simulink model "PWM_self_modified_PWM"  (R2022a)
settings: Solver=FixedStepAuto  StartTime=0.0  StopTime=stoptime  FixedStep=stepsize  MaxStep=2e-6  RelTol=1e-3
undefined symbols (not defined in the file or in its folder): Continuous, frequency, fs, gcbh, L, R, sps, sps_rtmsupport, spsSawtoothGeneratorModel, stepsize, u_sampletime, V, Vdc
libraries: spsIGBTDiodeLib x6, spsSeriesRLCBranchLib x3, spsGroundLib x1, spsThreePhaseVIMeasurementLib x1, spsDCVoltageSourceLib x1, spspowerguiLib x1
settings Model: Creator=Bob  LastModifiedBy=Bob

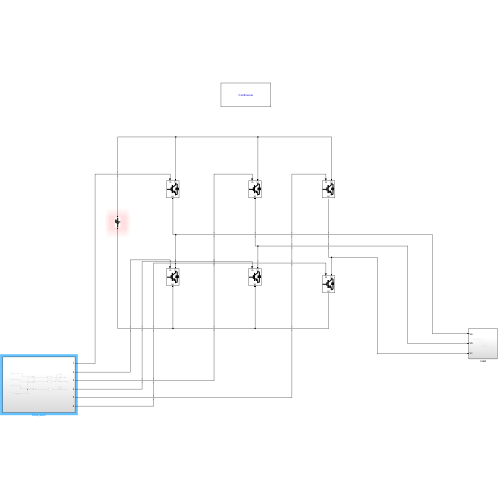
[thumbnail: Simulink's stored preview of the top-level diagram]
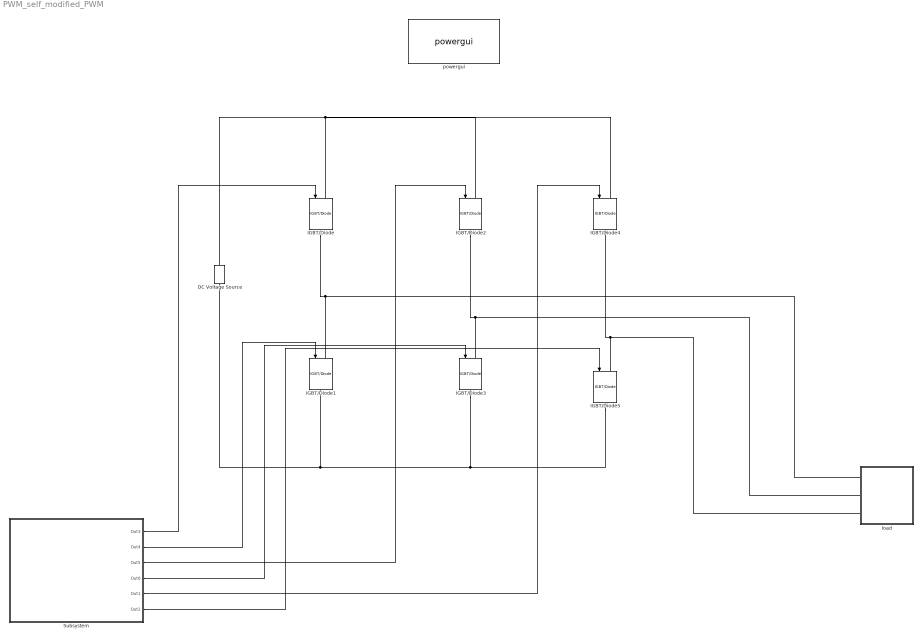
== system PWM_self_modified_PWM ==
  " load" : Subsystem
  DC Voltage Source : spsDCVoltageSourceLib/DC Voltage Source  Amplitude=Vdc  Measurements=None
  IGBT/Diode{,1..5} (6 alike) : spsIGBTDiodeLib/IGBT//Diode  Ron=1e-3  Rs=1e5  Cs=inf  Measurements=off
  Subsystem : Subsystem
  powergui : spspowerguiLib/powergui  Priority=1  SimulationMode=Continuous  SampleTime=stepsize  frequency=60  Iterations=50  frequencyindice=0  Pbase=100e6  ErrMax=1e-4  UnitsV=kV  UnitsW=MW  buscounter=0  FunctionMessages=off  echomessages=off  EnableUseOfTLC=off  CurrentSourceSwitches=off  DisableSnubberDevices=off  DisableRonSwitches=off  DisableVfSwitches=off  DisplayEquations=off  AutomaticDiscreteSolvers=off  SolverType=Tustin/Backward Euler (TBE)  Interpol=off  ExternalGateDelay=off  methode=off  Ts=100  x0status=blocks  SPID=on  SwTol=0  HookPort=off  NonlinearTolerance=1e-4  nMaxIteration=100  ContinueOnMaxIteration=off  RestoreLinks=warning  ResistiveCurrentMeasurement=off  Frange=[0:2:500]  Ylog=off  Xlog=on  ShowGrid=off  save=off  variable=ZData  structure=0  ZoomFFT=off  StartTime=0.0  cycles=1  DisplayStyle=1  fundamental=60  FreqAxis=off  MaxFrequency=1000  frequencyindicesteady=1  RmsSteady=1  display=off
  wires:
  Subsystem/1(Out3) -> IGBT/Diode/1
  Subsystem/2(Out4) -> IGBT/Diode1/1
  Subsystem/3(Out5) -> IGBT/Diode2/1
  Subsystem/4(Out6) -> IGBT/Diode3/1
  Subsystem/5(Out1) -> IGBT/Diode4/1
  Subsystem/6(Out2) -> IGBT/Diode5/1
  connections:
  IGBT/Diode4/LConn1 -- IGBT/Diode2/LConn1 -- IGBT/Diode/LConn1 -- DC Voltage Source/RConn1
  IGBT/Diode3/RConn1 -- IGBT/Diode5/RConn1 -- IGBT/Diode1/RConn1 -- DC Voltage Source/LConn1
  " load"/LConn2 -- IGBT/Diode3/LConn1 -- IGBT/Diode2/RConn1
  " load"/LConn1 -- IGBT/Diode1/LConn1 -- IGBT/Diode/RConn1
  " load"/LConn3 -- IGBT/Diode4/RConn1 -- IGBT/Diode5/LConn1

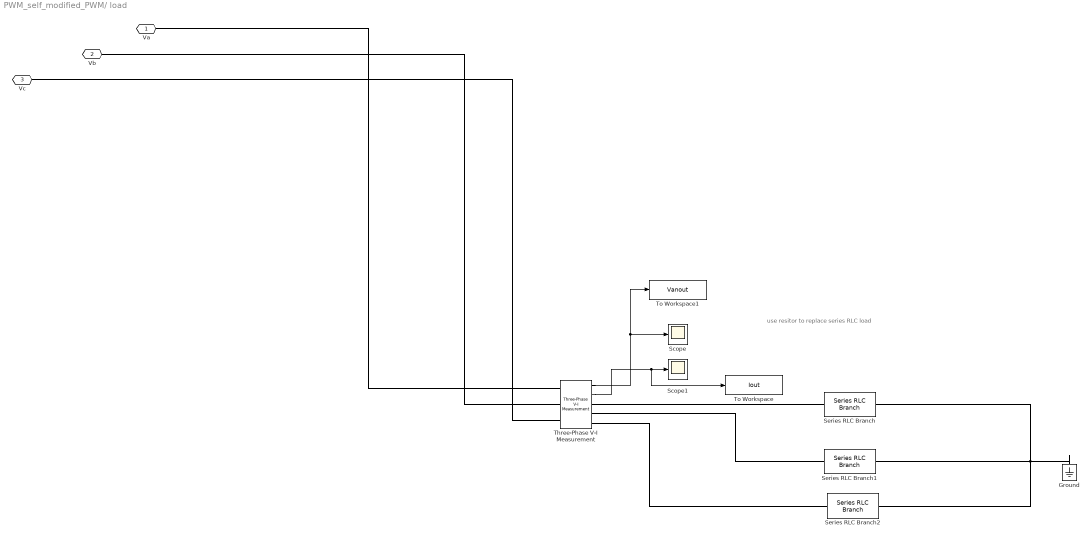
== system PWM_self_modified_PWM/ load ==
  note: use resitor to replace series RLC load
  Ground : spsGroundLib/Ground  LConnTagsString=a
  Scope : Scope
  Scope1 : Scope
  Series RLC Branch : spsSeriesRLCBranchLib/Series RLC Branch  LConnTagsString=__new0  RConnTagsString=__new0  BranchType=RL  Resistance=R  Inductance=L  SetiL0=off  InitialCurrent=0  Capacitance=1e-6  Setx0=off  InitialVoltage=0  Measurements=None
  Series RLC Branch1 : spsSeriesRLCBranchLib/Series RLC Branch  LConnTagsString=__new0  RConnTagsString=__new0  BranchType=RL  Resistance=R  Inductance=L  SetiL0=off  InitialCurrent=0  Capacitance=1e-6  Setx0=off  InitialVoltage=0  Measurements=None
  Series RLC Branch2 : spsSeriesRLCBranchLib/Series RLC Branch  LConnTagsString=__new0  RConnTagsString=__new0  BranchType=RL  Resistance=R  Inductance=L  SetiL0=off  InitialCurrent=0  Capacitance=1e-6  Setx0=off  InitialVoltage=0  Measurements=None
  Three-Phase V-I Measurement : spsThreePhaseVIMeasurementLib/Three-Phase V-I Measurement  VoltageMeasurement=phase-to-ground  SetLabelV=off  LabelV=Vabc  Vpu=off  VpuLL=off  CurrentMeasurement=yes  SetLabelI=off  LabelI=Iabc  Ipu=off  Pbase=100e6  Vbase=500e3  OutputType=Complex  PhasorSimulation=off  PSBequivalent=0
  To Workspace : ToWorkspace  VariableName=Iout  SampleTime=-1
      settings: Save2DSignal=2-D array (concatenate along first dimension)
  To Workspace1 : ToWorkspace  VariableName=Vanout  SampleTime=-1
      settings: Save2DSignal=2-D array (concatenate along first dimension)
  Va : PMIOPort  Side=Left
  Vb : PMIOPort  Port=2  Side=Left
  Vc : PMIOPort  Port=3  Side=Left
  wires:
  Three-Phase V-I Measurement/2 -> To Workspace/1, Scope1/1
  Three-Phase V-I Measurement/1 -> Scope/1, To Workspace1/1
  connections:
  Three-Phase V-I Measurement/LConn2 -- Vb/RConn1
  Three-Phase V-I Measurement/LConn3 -- Vc/RConn1
  Three-Phase V-I Measurement/LConn1 -- Va/RConn1
  Ground/LConn1 -- Series RLC Branch2/RConn1 -- Series RLC Branch1/RConn1 -- Series RLC Branch/RConn1
  Series RLC Branch/LConn1 -- Three-Phase V-I Measurement/RConn1
  Series RLC Branch1/LConn1 -- Three-Phase V-I Measurement/RConn2
  Series RLC Branch2/LConn1 -- Three-Phase V-I Measurement/RConn3

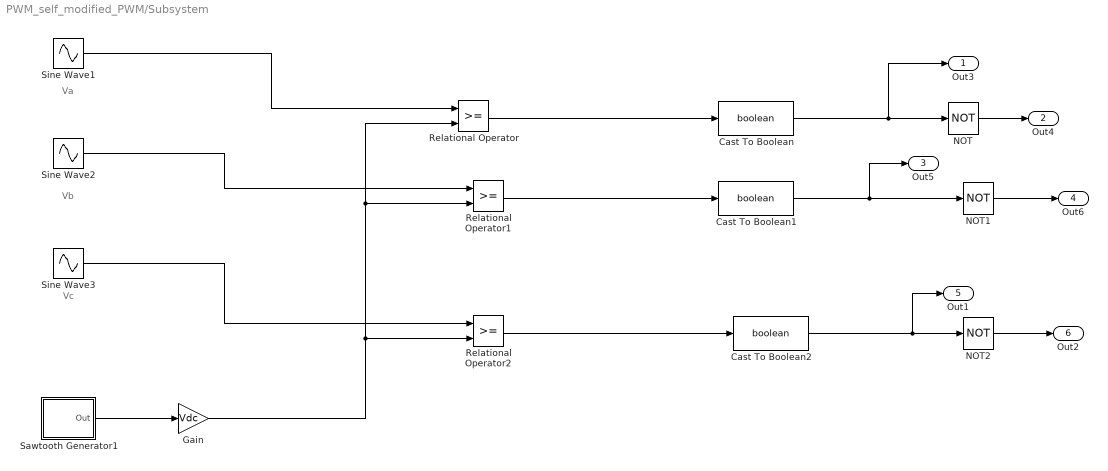
== system PWM_self_modified_PWM/Subsystem ==
  note: Vb
  note: Vc
  note: Va
  Cast To Boolean : DataTypeConversion  OutDataTypeStr=boolean  SaturateOnIntegerOverflow=off  RndMeth=Floor
  Cast To Boolean1 : DataTypeConversion  OutDataTypeStr=boolean  SaturateOnIntegerOverflow=off  RndMeth=Floor
  Cast To Boolean2 : DataTypeConversion  OutDataTypeStr=boolean  SaturateOnIntegerOverflow=off  RndMeth=Floor
  Gain : Gain  Gain=Vdc
  NOT : Logic  Operator=NOT  IconShape=distinctive  AllPortsSameDT=off  OutDataTypeStr=boolean
  NOT1 : Logic  Operator=NOT  IconShape=distinctive  AllPortsSameDT=off  OutDataTypeStr=boolean
  NOT2 : Logic  Operator=NOT  IconShape=distinctive  AllPortsSameDT=off  OutDataTypeStr=boolean
  Relational Operator : RelationalOperator  OutDataTypeStr=boolean  RndMeth=Simplest  InputSameDT=off
  Relational Operator1 : RelationalOperator  OutDataTypeStr=boolean  RndMeth=Simplest  InputSameDT=off
  Relational Operator2 : RelationalOperator  OutDataTypeStr=boolean  RndMeth=Simplest  InputSameDT=off
  Sawtooth Generator1 : Subsystem  AncestorBlock=spsSawtoothGeneratorLib/Sawtooth Generator  DialogController=POWERSYS.PowerSysDialog  LoadFcn=sps_rtmsupport('LoadFcn', gcbh);  StartFcn=sps_rtmsupport('StartFcn', gcbh);  StopFcn=sps_rtmsupport('StopFcn', gcbh);  mask(Sawtooth Generator){Freq=fs, Phase=0, Ts=0}
      mask prompts: Freq "Frequency (Hz):"; Phase "Phase (degrees):"; Ts "Sample time:"
      mask help: Generate a sawtooth wave with peak of -1 to +1.
      mask init:
      | block = gcb;
      | [WantBlockChoice,Ts,sps] = powericon('SawtoothGeneratorInit',block,Phase,Freq,Ts);
      | powericon('SetInternalModels','set',block,WantBlockChoice);
      settings: CopyFcn=sps_rtmsupport('CopyFcn', gcbh);  DeleteFcn=sps_rtmsupport('DeleteFcn', gcbh);  UndoDeleteFcn=sps_rtmsupport('UndoDeleteFcn', gcbh);  ModelCloseFcn=sps_rtmsupport('ModelCloseFcn', gcbh);  PreSaveFcn=sps_rtmsupport('PreSaveFcn', gcbh);  PostSaveFcn=sps_rtmsupport('PostSaveFcn', gcbh);  NameChangeFcn=sps_rtmsupport('NameChangeFcn', gcbh);  PreCopyFcn=sps_rtmsupport('PreCopyFcn', gcbh);  OpenFcn=sps_rtmsupport('OpenFcn', gcbh, []);  CloseFcn=sps_rtmsupport('CloseFcn', gcbh);  PreDeleteFcn=sps_rtmsupport('PreDeleteFcn', gcbh);
      mask Help: helpview(psbhelp);
      mask Display: plot([sps.time sps.time+sps.time(end)],repmat(sps.Out,1,2))
  Sine Wave1 : Sin  Amplitude=V  Frequency=2*pi*frequency  SampleTime=0
  Sine Wave2 : Sin  Amplitude=V  Frequency=2*pi*frequency  Phase=-2*pi/3  SampleTime=0
  Sine Wave3 : Sin  Amplitude=V  Frequency=2*pi*frequency  Phase=-4*pi/3  SampleTime=0
  Out3 : Outport
  Out4 : Outport  Port=2
  Out5 : Outport  Port=3
  Out6 : Outport  Port=4
  Out1 : Outport  Port=5
  Out2 : Outport  Port=6
  wires:
  Relational Operator2/1 -> Cast To Boolean2/1
  Cast To Boolean/1 -> Out3/1, NOT/1
  Sine Wave1/1 -> Relational Operator/1
  Gain/1 -> Relational Operator2/2, Relational Operator1/2, Relational Operator/2
  Relational Operator/1 -> Cast To Boolean/1
  Sawtooth Generator1/1(Out) -> Gain/1
  Sine Wave2/1 -> Relational Operator1/1
  Relational Operator1/1 -> Cast To Boolean1/1
  Sine Wave3/1 -> Relational Operator2/1
  Cast To Boolean1/1 -> Out5/1, NOT1/1
  Cast To Boolean2/1 -> Out1/1, NOT2/1
  NOT/1 -> Out4/1
  NOT1/1 -> Out6/1
  NOT2/1 -> Out2/1

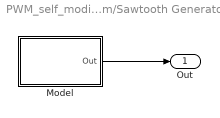
== system PWM_self_modified_PWM/Subsystem/Sawtooth Generator1 ==
  Model : Subsystem  AncestorBlock=spsSawtoothGeneratorModel/Continuous
  Out : Outport  VectorParamsAs1DForOutWhenUnconnected=off
  wires:
  Model/1(Out) -> Out/1

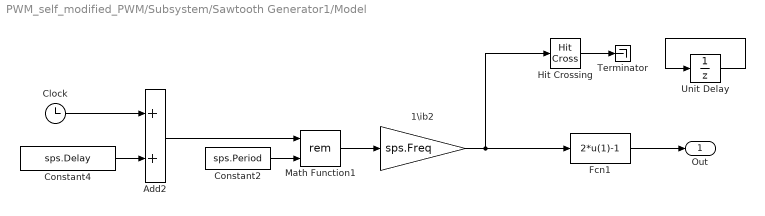
== system PWM_self_modified_PWM/Subsystem/Sawtooth Generator1/Model ==
  1\ib2 : Gain  Gain=sps.Freq  SaturateOnIntegerOverflow=on  OutDataTypeStr=Inherit: Same as input  ParamDataTypeStr=Inherit: Same as input
  Add2 : Sum
  Clock : Clock
  Constant2 : Constant  Value=sps.Period  SampleTime=0
  Constant4 : Constant  Value=sps.Delay  SampleTime=0
  Fcn1 : Fcn  Expr=2*u(1)-1
  Hit Crossing : HitCross
  Math Function1 : Math  Operator=rem  SignedPower=on
  Terminator : Terminator
  Unit Delay : UnitDelay  SampleTime=u_sampletime  HasFrameUpgradeWarning=on
  Out : Outport
  wires:
  Hit Crossing/1 -> Terminator/1
  1\ib2/1 -> Fcn1/1, Hit Crossing/1
  Fcn1/1 -> Out/1
  Unit Delay/1 -> Unit Delay/1
  Add2/1 -> Math Function1/1
  Constant4/1 -> Add2/2
  Constant2/1 -> Math Function1/2
  Clock/1 -> Add2/1
  Math Function1/1 -> 1\ib2/1
